simulink model "compass_servo"  (Simulink 6.4)
settings: Solver=ode45  StartTime=0.0  StopTime=10.0  RelTol=1e-3
libraries: simulink x2
settings Model: LastModifiedBy=jporter

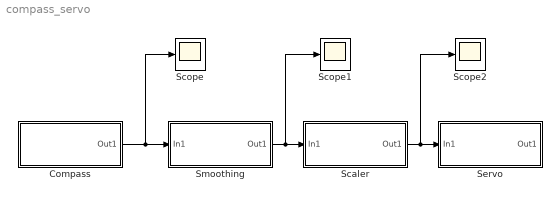
== system compass_servo ==
  Compass : Subsystem
  Scaler : Subsystem
  Scope : Scope
      settings: YMin=0  YMax=3600
  Scope1 : Scope
      settings: YMin=0  YMax=3600
  Scope2 : Scope
      settings: YMin=1000  YMax=8000  SaveName=ScopeData2
  Servo : Subsystem
  Smoothing : Subsystem
  wires:
  Compass/1(Out1) -> Smoothing/1(In1), Scope/1
  Smoothing/1(Out1) -> Scaler/1(In1), Scope1/1
  Scaler/1(Out1) -> Servo/1(In1), Scope2/1

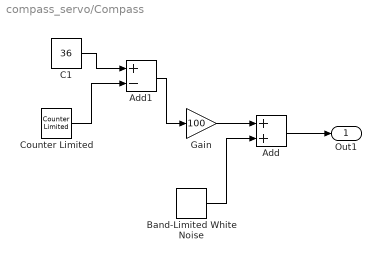
== system compass_servo/Compass ==
  Add : Sum  OutScaling=2^-10
  Add1 : Sum  Inputs=+-  OutScaling=2^-10
  Band-Limited White Noise : simulink/Sources/Band-Limited White Noise  SystemSampleTime=-1  Cov=[500]  Ts=1/8  seed=[23341]
  C1 : Constant  Value=36  OutDataType=sfix(16)  ConRadixGroup=Use specified scaling  OutScaling=2^0  SampleTime=inf  FramePeriod=inf
  Counter Limited : simulink/Sources/Counter Limited  SystemSampleTime=-1  uplimit=36  tsamp=1/8
  Gain : Gain  Gain=100
  Out1 : Outport
  wires:
  Add/1 -> Out1/1
  Band-Limited White Noise/1 -> Add/2
  Gain/1 -> Add/1
  C1/1 -> Add1/1
  Counter Limited/1 -> Add1/2
  Add1/1 -> Gain/1

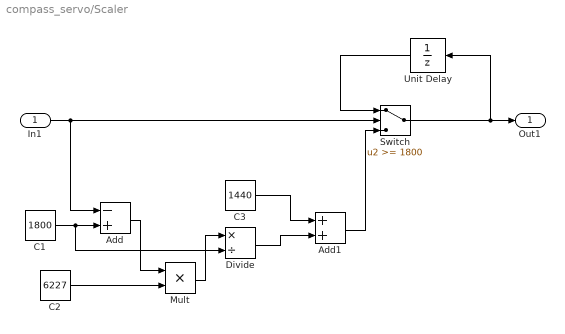
== system compass_servo/Scaler ==
  In1 : Inport
  Add : Sum  Inputs=-+  OutScaling=2^-10
  Add1 : Sum  OutScaling=2^-10
  C1 : Constant  Value=1800  OutDataType=sfix(16)  ConRadixGroup=Use specified scaling  OutScaling=2^0  SampleTime=inf  FramePeriod=inf
  C2 : Constant  Value=6227  OutDataType=sfix(16)  ConRadixGroup=Use specified scaling  OutScaling=2^0  SampleTime=inf  FramePeriod=inf
  C3 : Constant  Value=1440  OutDataType=sfix(16)  ConRadixGroup=Use specified scaling  OutScaling=2^0  SampleTime=inf  FramePeriod=inf
  Divide : Product  Inputs=*/  OutScaling=2^-10
  Mult : Product  Inputs=**  OutScaling=2^-10
  Switch : Switch  Threshold=1800
  Unit Delay : UnitDelay  Orientation=left  X0=1440  SampleTime=-1
  Out1 : Outport
  wires:
  In1/1 -> Add/1, Switch/2
  C1/1 -> Add/2, Divide/2
  Add/1 -> Mult/1
  C2/1 -> Mult/2
  Mult/1 -> Divide/1
  C3/1 -> Add1/1
  Divide/1 -> Add1/2
  Switch/1 -> Out1/1, Unit Delay/1
  Unit Delay/1 -> Switch/1
  Add1/1 -> Switch/3

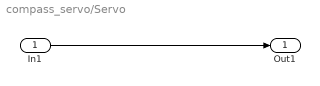
== system compass_servo/Servo ==
  In1 : Inport
  Out1 : Outport
  wires:
  In1/1 -> Out1/1

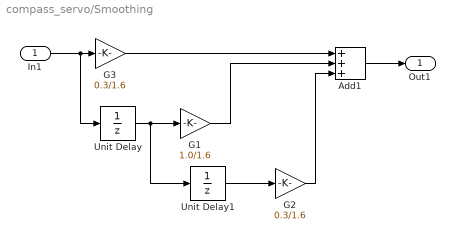
== system compass_servo/Smoothing ==
  In1 : Inport
  Add1 : Sum  Inputs=+++  OutScaling=2^-10
  G1 : Gain  Gain=1.0/1.6
  G2 : Gain  Gain=0.3/1.6
  G3 : Gain  Gain=0.3/1.6
  Unit Delay : UnitDelay  SampleTime=-1
  Unit Delay1 : UnitDelay  SampleTime=-1
  Out1 : Outport
  wires:
  In1/1 -> G3/1, Unit Delay/1
  G3/1 -> Add1/1
  Unit Delay/1 -> G1/1, Unit Delay1/1
  G1/1 -> Add1/2
  Unit Delay1/1 -> G2/1
  G2/1 -> Add1/3
  Add1/1 -> Out1/1
